simulink model "dual500MHzPFB"  (Simulink 6.2)
settings: Solver=ode45  StartTime=0.0  StopTime=10000  RelTol=1e-3
libraries: xbsIndex_r3 x2070, casper_library x180, xps_library x12, gtkWave x5, gavrt_library x1
(part 11 of 20)

== system dual500MHzPFB/cfgspec/PFB_Subsystem/pfb_fir_real1/pol1_in1_first_tap/pfb_coeff_gen ==
  din : Inport  Port=1  LatchInput=off
  sync : Inport  Port=2  LatchInput=off
  Concat : xbsIndex_r3/Concat  num_inputs=2  explicit_period=off  period=1  dbl_ovrd=off
  Counter : xbsIndex_r3/Counter  cnt_type=Free Running  n_bits=8  bin_pt=0  arith_type=Unsigned  start_count=0  cnt_to=Inf  cnt_by_val=1  operation=Up  explicit_period=on  period=1  load_pin=off  rst=on  en=off  dbl_ovrd=off  show_param=off  use_rpm=on  gen_core=off
      settings: xl_area=[0, 0, 0, 0, 0, 0, 0]
  Delay : xbsIndex_r3/Delay  latency=bram_latency+1  reg_retiming=off  explicit_period=off  period=1  en=off  accept_only_valid=off  init_zero=on  dbl_ovrd=off  show_param=off
      settings: xl_area=[0, 0, 0, 0, 0, 0, 0]
  Delay1 : xbsIndex_r3/Delay  latency=3  reg_retiming=off  explicit_period=off  period=1  en=off  accept_only_valid=off  init_zero=on  dbl_ovrd=off  show_param=off
      settings: xl_area=[0, 0, 0, 0, 0, 0, 0]
  ROM1 : xbsIndex_r3/ROM  depth=256  initVector=[3.1185374660155e-018 0.000313853577146838 0.000630949867739494 0.000952101185429728 0.00127813150918155 0.00160987609990742 0.00194818110908897 0.00229390317955257 0.00264790903857445 0.00301107508349448 0.00338428696002226 0.00376843913342326 0.00416443445277708 0.00457318370850389 0.00499560518335912 0.00543262419710063 0.00588517264503594 0.00635418853066137 0.00684061549260819 0.00734540232611445 0.00786950249924483 0.00841387366408389 0.0089794771631314 0.00956727753113161 0.0101782419925713 0.010813339955084 0.0114735424990016 0.0121598218632949 0.0128731509281507 0.0136145026944319 0.014384849760272 0.0151851637950551 0.0160164150110379 0.0168795716328685 0.0177755993652613 0.0187054608590871 0.0196701151761411 0.0206705172528497 0.0217076173631834 0.0227823605810373 0.023895686242349 0.0250485274072193 0.0262418103223038 0.027476453883745 0.0287533691009129 0.0300734585612245 0.031437615896311 0.0328467252498039 0.0343016607470079 0.0358032859667318 0.0373524534155453 0.0389500040047317 0.0405967665302039 0.042293557155651 0.044041178899183 0.0458404211237378 0.0476920590315163 0.0495968531627079 0.0515555488987685 0.0535688759705108 0.0556375479712659 0.0577622618753727 0.0599436975622499 0.0621825173463032 0.0644793655129179 0.0668348678607861 0.0692496312508128 0.0717242431618448 0.0742592712534627 0.0768552629360733 0.0795127449485372 0.0822322229435622 0.0850141810810928 0.0878590816299174 0.0907673645777188 0.0937394472497809 0.0967757239365713 0.0998765655304047 0.103042319171399 0.106273307902919 0.109569830336718 0.112932160327956 0.116360546660299 0.119855212741273 0.123416356308059 0.127044149143908 0.13073873680534 0.134500238360297 0.138328746137415 0.142224325486561 0.146187014550802 0.15021682404994 0.154313737075755 0.158477708899094 0.162708666788946 0.167006509843603 0.171371108834052 0.175802306059696 0.180299915216515 0.184863721277773 0.189493480387363 0.194188919765877 0.198949737629496 0.203775603121767 0.208666156258342 0.213621007884754 0.218639739647272 0.22372190397691 0.228867024086619 0.234074593981714 0.239344078483567 0.244674913266598 0.250066504908579 0.255518230954276 0.261029439992432 0.266599451746097 0.272227557176302 0.277913018599066 0.283655069815719 0.289452916256518 0.29530573513754 0.301212675630786 0.307172859047495 0.313185379034582 0.31924930178417 0.325363666256144 0.331527484413666 0.33773974147157 0.343999396157563 0.350305380986143 0.356656602545143 0.363051941794802 0.369490254379254 0.375970370950336 0.382491097503579 0.389051215726279 0.395649483357505 0.402284634559911 0.40895538030322 0.415660408759225 0.422398385708151 0.429167954956233 0.435967738764334 0.44279633828744 0.449652334024857 0.456534286280925 0.46344073563607 0.470370203428 0.477321192242848 0.484292186416068 0.491281652542864 0.498288039997961 0.505309781464482 0.512345293471729 0.51939297694163 0.526451217743632 0.533518387257796 0.540592842945872 0.547672928930096 0.55475697657947 0.56184330510328 0.568930222151592 0.576016024422464 0.583098998275629 0.590177420352365 0.597249558201307 0.604313670909903 0.611368009741263 0.61841081877612 0.625440335559606 0.632454791752587 0.639452413787252 0.64643142352668 0.653390038928083 0.660326474709457 0.667238943019316 0.67412565410924 0.68098481700893 0.68781464020346 0.694613332312453 0.701379102770851 0.708110162510993 0.714804724645695 0.721461005152022 0.728077223555458 0.734651603614152 0.741182374002953 0.747667768996907 0.754106029153935 0.760495401996357 0.766834142690977 0.773120514727421 0.779352790594407 0.785529252453665 0.79164819281118 0.797707915185476 0.803706734772626 0.809642979107687 0.815514988722272 0.821321117797946 0.827059734815166 0.832729223197448 0.838327981950501 0.843854426296004 0.849306988299761 0.854684117493933 0.859984281493085 0.865205966603733 0.870347678427156 0.875407942455152 0.880385304658511 0.885278332067902 0.890085613346922 0.894805759357052 0.899437403714244 0.903979203336905 0.908429838985005 ...(+699 chars)]  arith_type="Signed  (2's comp)"  n_bits=8  bin_pt=7  latency=2  init_zero=on  explicit_period=off  period=1  rst=off  init_reg=0  en=off  dbl_ovrd=off  show_param=on  distributed_mem=off  use_rpm=on  gen_core=off
      settings: xl_area=[0, 0, 0, 0, 0, 0, 0]
  ROM2 : xbsIndex_r3/ROM  depth=256  initVector=[0.999999458258868 0.999931021245783 0.999743065596651 0.999435647723483 0.999008859879318 0.998462830120572 0.997797722254753 0.997013735773593 0.996111105771608 0.995090102850134 0.993951033006882 0.992694237511061 0.991320092764127 0.989829010146224 0.988221435848383 0.986497850690571 0.984658769925647 0.982704743029348 0.980636353476378 0.978454218502709 0.976158988854215 0.97375134852174 0.971232014462726 0.968601736309539 0.96586129606462 0.963011507782594 0.960053217239501 0.956987301589287 0.953814669007724 0.950536258323912 0.947153038639539 0.943666008936081 0.940076197670108 0.936384662356893 0.932592489142517 0.928700792364653 0.924710714102252 0.920623423714318 0.916440117367999 0.912162017556199 0.907790372604941 0.903326456170708 0.89877156672798 0.894127027047217 0.889394183663526 0.884574406336234 0.879669087499654 0.874679641705254 0.869607505055511 0.864454134629704 0.859221007901897 0.853909622151394 0.848521493865925 0.843058158137836 0.837521168053561 0.831912094076659 0.826232523424682 0.820484059440178 0.814668320956092 0.80878694165588 0.802841569428602 0.796833865719299 0.790765504874954 0.784638173486316 0.778453569725904 0.77221340268248 0.765919391692288 0.759573265667376 0.753176762421293 0.746731627992459 0.740239615965535 0.733702486791073 0.727122007103769 0.720499949039619 0.713838089552282 0.707138209728965 0.700402094106126 0.693631529985308 0.686828306749403 0.679994215179664 0.673131046773749 0.666240593065125 0.659324644944108 0.65238499198086 0.645423421750641 0.6384417191616 0.63144166578542 0.624425039191102 0.617393612282178 0.610349152637658 0.603293421856988 0.596228174909311 0.589155159487311 0.58207611536593 0.574992773766228 0.567906856724672 0.560820076468121 0.55373413479477 0.546650722461346 0.539571518576789 0.532498190002693 0.525432390760777 0.518375761447603 0.511329928656835 0.504296504409245 0.497277085590735 0.490273253398593 0.483286572796234 0.476318591976636 0.469370841834709 0.462444835448811 0.455542067571624 0.448664014130602 0.441812131738202 0.434987857212088 0.428192607105504 0.421427777248019 0.414694742296809 0.407994855298675 0.401329447262956 0.39469982674551 0.388107279443932 0.381553067804161 0.37503843063862 0.368564582756054 0.362132714603191 0.355743991918358 0.349399555397198 0.343100520370588 0.336847976494894 0.330642987454655 0.324486590677818 0.318379797063608 0.31232359072313 0.306318928732789 0.300366740900606 0.2944679295455 0.288623369289612 0.282833906863717 0.277100360925787 0.271423521892756 0.265804151785514 0.260242984087177 0.254740723614657 0.249298046403554 0.243915599606379 0.238594001404134 0.233333840931226 0.228135678213734 0.22300004412101 0.217927440330587 0.212918339306393 0.207973184290218 0.203092389306419 0.198276339179798 0.193525389566635 0.188839866998784 0.184220068940809 0.179666263860066 0.175178691309668 0.170757562024254 0.166403058028479 0.162115332758128 0.157894511193761 0.153740690006788 0.149653937717859 0.145634294867461 0.141681774198606 0.137796360851467 0.13397801256985 0.130226659919365 0.126542206517129 0.122924529272895 0.119373478641418 0.115888878885919 0.112470528352485 0.10911819975523 0.105831640472054 0.102610572850808 0.0994546945257127 0.0963636787438044 0.0933371747012584 0.0903748078893658 0.0874761804499801 0.0846408715402248 0.0818684377062569 0.0791584132658749 0.0765103106997557 0.0739236210511041 0.0713978143334908 0.0689323399466543 0.0665266271000393 0.0641800852438365 0.0618921045072929 0.0596620561440508 0.0574892929842778 0.0553731498933419 0.0533129442367877 0.0513079763513631 0.0493575300218483 0.0474608729634309 0.045617257309375 0.0438259201037253 0.0420860837987887 0.0403969567571315 0.0387577337578319 0.0371675965067231 0.0356257141503632 0.0341312437934655 0.0326833310195229 0.031281110414359 0.0299237060923366 0.0286102322249562 0.0273397935715735 0.0261114860119683 0.0249243970804927 0.0237776065015307 0.0226701867259983 0.0216012034686154 0.0205697162456796 0.019574778913074 ...(+681 chars)]  arith_type="Signed  (2's comp)"  n_bits=8  bin_pt=7  latency=2  init_zero=on  explicit_period=off  period=1  rst=off  init_reg=0  en=off  dbl_ovrd=off  show_param=on  distributed_mem=off  use_rpm=on  gen_core=off
      settings: xl_area=[0, 0, 0, 0, 0, 0, 0]
  Register : xbsIndex_r3/Register  init=0  reg_only_valid=off  explicit_period=off  period=1  rst=off  en=off  out_en=off  dbl_ovrd=off  show_param=off
      settings: xl_area=[0, 0, 0, 0, 0, 0, 0]
  Reinterpret1 : xbsIndex_r3/Reinterpret  force_arith_type=on  arith_type=Unsigned  force_bin_pt=on  bin_pt=0  force_valid=on
  Reinterpret2 : xbsIndex_r3/Reinterpret  force_arith_type=on  arith_type=Unsigned  force_bin_pt=on  bin_pt=0  force_valid=on
  dout : Outport
  sync_out : Outport  Port=2
  coeff : Outport  Port=3
  wires:
  din/1 -> Delay1/1
  Delay1/1 -> dout/1
  sync/1 -> Counter/1, Delay/1
  Delay/1 -> sync_out/1
  Concat/1 -> Register/1
  Register/1 -> coeff/1
  Counter/1 -> ROM1/1, ROM2/1
  ROM1/1 -> Reinterpret1/1
  Reinterpret1/1 -> Concat/1
  ROM2/1 -> Reinterpret2/1
  Reinterpret2/1 -> Concat/2

== system dual500MHzPFB/cfgspec/PFB_Subsystem/pfb_fir_real1/pol1_in1_last_tap/pfb_real_add_tree ==
  din : Inport  Port=1  LatchInput=off
  sync : Inport  Port=2  LatchInput=off
  Reint0 : xbsIndex_r3/Reinterpret  force_arith_type=on  arith_type="Signed  (2's comp)"  force_bin_pt=on  bin_pt=CoeffBitWidth + BitWidthIn - 2  force_valid=on
  Reint1 : xbsIndex_r3/Reinterpret  force_arith_type=on  arith_type="Signed  (2's comp)"  force_bin_pt=on  bin_pt=CoeffBitWidth + BitWidthIn - 2  force_valid=on
  Slice0 : xbsIndex_r3/Slice  mode=Upper Bit Location + Width  nbits=CoeffBitWidth + BitWidthIn  bit1=-0*(CoeffBitWidth + BitWidthIn)  base1=MSB of Input  bit0=0  base0=MSB of Input  boolean_output=off  explicit_period=off  period=1  dbl_ovrd=off
  Slice1 : xbsIndex_r3/Slice  mode=Upper Bit Location + Width  nbits=CoeffBitWidth + BitWidthIn  bit1=-1*(CoeffBitWidth + BitWidthIn)  base1=MSB of Input  bit0=0  base0=MSB of Input  boolean_output=off  explicit_period=off  period=1  dbl_ovrd=off
  adder_tree1 : Subsystem  AncestorBlock=casper_library/Misc/adder_tree  mask(adder_tree){n_inputs=2, latency=2}
      mask prompts: n_inputs "Number of Inputs"; latency "Add Latency"
      mask help: Sums all inputs using a tree of adds and delays.
      mask init:
      | adder_tree_init(gcb, ...
      |     'n_inputs', n_inputs, ...
      |     'latency', latency);
      settings: AttributesFormatString=latency 2
      mask Help: eval('xlWeb([getenv(''MLIB_ROOT''), ''\doc\html\sp_adder_tree\sp_adder_tree.html''])')
  convert1 : xbsIndex_r3/Convert  arith_type="Signed  (2's comp)"  n_bits=BitWidthOut  bin_pt=BitWidthOut-1  quantization=Truncate  overflow=Saturate  latency=add_latency  explicit_period=off  period=1  dbl_ovrd=off  show_param=off  inserted_by_tool=off  pipeline=off
      settings: xl_area=[0, 0, 0, 0, 0, 0, 0]
  delay1 : xbsIndex_r3/Delay  latency=2  reg_retiming=off  explicit_period=off  period=1  en=off  accept_only_valid=off  init_zero=on  dbl_ovrd=off  show_param=off
      settings: xl_area=[0, 0, 0, 0, 0, 0, 0]
  scale1 : xbsIndex_r3/Scale  scale_factor=-2  explicit_period=off  period=1  dbl_ovrd=off
  dout : Outport
  sync_out : Outport  Port=2
  wires:
  adder_tree1/2(dout) -> scale1/1
  scale1/1 -> convert1/1
  convert1/1 -> dout/1
  sync/1 -> adder_tree1/1(sync)
  adder_tree1/1(sync_out) -> delay1/1
  delay1/1 -> sync_out/1
  din/1 -> Slice0/1, Slice1/1
  Slice0/1 -> Reint0/1
  Reint0/1 -> adder_tree1/2(din1)
  Slice1/1 -> Reint1/1
  Reint1/1 -> adder_tree1/3(din2)

== system dual500MHzPFB/cfgspec/PFB_Subsystem/pfb_fir_real1/pol1_in2_first_tap/delay ==
  In1 : Inport  Port=1  LatchInput=off
  delay_bram : casper_library/Delays/delay_bram  DelayLen=2^(PFBSize-n_inputs)  bram_latency=bram_latency
  Out1 : Outport
  wires:
  In1/1 -> delay_bram/1
  delay_bram/1 -> Out1/1

== system dual500MHzPFB/cfgspec/PFB_Subsystem/pfb_fir_real1/pol1_in2_first_tap/pfb_coeff_gen ==
  din : Inport  Port=1  LatchInput=off
  sync : Inport  Port=2  LatchInput=off
  Concat : xbsIndex_r3/Concat  num_inputs=2  explicit_period=off  period=1  dbl_ovrd=off
  Counter : xbsIndex_r3/Counter  cnt_type=Free Running  n_bits=8  bin_pt=0  arith_type=Unsigned  start_count=0  cnt_to=Inf  cnt_by_val=1  operation=Up  explicit_period=on  period=1  load_pin=off  rst=on  en=off  dbl_ovrd=off  show_param=off  use_rpm=on  gen_core=off
      settings: xl_area=[0, 0, 0, 0, 0, 0, 0]
  Delay : xbsIndex_r3/Delay  latency=bram_latency+1  reg_retiming=off  explicit_period=off  period=1  en=off  accept_only_valid=off  init_zero=on  dbl_ovrd=off  show_param=off
      settings: xl_area=[0, 0, 0, 0, 0, 0, 0]
  Delay1 : xbsIndex_r3/Delay  latency=3  reg_retiming=off  explicit_period=off  period=1  en=off  accept_only_valid=off  init_zero=on  dbl_ovrd=off  show_param=off
      settings: xl_area=[0, 0, 0, 0, 0, 0, 0]
  ROM1 : xbsIndex_r3/ROM  depth=256  initVector=[7.82033640873917e-005 0.000392792117321438 0.00071082554813207 0.00103311892199487 0.00136049907461725 0.00169380402655518 0.00203388258985642 0.00238159396690193 0.00273780734162119 0.00310340146326166 0.00347926422289714 0.00386629222286377 0.00426539033931678 0.00467747127810509 0.00510345512416486 0.00554426888463693 0.00600084602591724 0.00647412600485223 0.00696505379429587 0.00747457940324748 0.00800365739179369 0.00855324638108065 0.00912430855854599 0.00971780917864314 0.0103347160592936 0.0109759990743052 0.0116426296419981 0.0123355802102817 0.0130558237384286 0.0138043331757953 0.0145820809377384 0.0153900383789824 0.0162291752646908 0.0171004592395002 0.0180048552947743 0.0189433252343389 0.0199168271389599 0.0209263148298273 0.021972737331309 0.0230570383332419 0.0241801556530246 0.0253430206977808 0.0265465579268609 0.0277916843149512 0.0290793088160584 0.0304103318286413 0.0317856446621574 0.0332061290052946 0.0346726563961596 0.0361860876946888 0.0377472725575551 0.0393570489158354 0.0410162424557095 0.0427256661024564 0.0444861195080145 0.046298388542371 0.0481632447890453 0.0500814450449274 0.0520537308247352 0.0540808278703483 0.0561634456652778 0.0583022769545272 0.0604979972700995 0.0627512644624029 0.0650627182378034 0.067432979702574 0.0698626509134837 0.07235231443527 0.0749025329052334 0.0775138486051921 0.0801867830410294 0.082921836530065 0.0857194877964775 0.0885801935750023 0.0915043882231255 0.0944924833419901 0.0975448674062286 0.100661905402931 0.103843938479953 0.107091283603769 0.110404233227058 0.113783054966233 0.117227991289079 0.120739259212706 0.124317050011981 0.127961528938623 0.131672834951122 0.135451080455663 0.139296351058194 0.143208705327813 0.147188174571609 0.151234762621111 0.155348445630488 0.159529171886614 0.163776861631156 0.168091406894782 0.172472671343625 0.176920490138103 0.18143466980421 0.186014988117371 0.190661193998959 0.195373007425566 0.200150119351105 0.204992191641821 0.209898857024285 0.214869719046434 0.219904352051709 0.225002301166354 0.230163082299916 0.235386182158984 0.240671058274206 0.2460171390406 0.251423823771201 0.256890482764031 0.262416457382418 0.26800106014867 0.273643574851073 0.279343256664236 0.285099332282737 0.290911000068066 0.296777430208813 0.302697764894093 0.308671118500132 0.314696577789995 0.320773202126374 0.326900023697389 0.333076047755331 0.339300252868267 0.345571591184427 0.351888988709288 0.358251345595259 0.364657536443868 0.37110641062034 0.377596792580462 0.384127482209607 0.390697255173799 0.397304863282687 0.40394903486429 0.41062847515137 0.417341866679289 0.424087869695195 0.430865122578368 0.437672242271578 0.444507824723272 0.451370445340415 0.458258659451806 0.46517100278169 0.472105991933451 0.479062124883217 0.486037881483159 0.493031723974274 0.50004209750845 0.507067430679598 0.514106136063612 0.521156610766955 0.528217236983621 0.535286382560249 0.542362401569151 0.549443634889005 0.556528410792964 0.563615045543947 0.570701843996833 0.577787100207321 0.584869098047179 0.591946111825632 0.599016406916601 0.606078240391542 0.613129861657594 0.620169513100771 0.627195430733905 0.634205844849072 0.641198980674199 0.648173059033581 0.655126297012004 0.662056908622189 0.668963105475262 0.675843097453958 0.682695093388247 0.6895173017331 0.696307931248092 0.703065191678525 0.709787294437785 0.716472453290627 0.723118885037072 0.729724810196624 0.736288453692496 0.742808045535534 0.749281821507542 0.755708023843698 0.762084901913749 0.768410712901686 0.774683722483594 0.780902205503364 0.787064446645969 0.793168741108002 0.799213395265163 0.805196727336407 0.811117068044443 0.816972761272283 0.822762164715558 0.828483650530292 0.834135605975834 0.839716434052685 0.84522455413489 0.850658402596745 0.856016433433509 0.861297118875845 0.866498949997721 0.871620437317469 0.876660111391761 0.881616523402199 0.886488245734271 0.891273872548405 0.89597202034285 0.900581328508143 0.905100459872888 0.909528101240623 ...(+701 chars)]  arith_type="Signed  (2's comp)"  n_bits=8  bin_pt=7  latency=2  init_zero=on  explicit_period=off  period=1  rst=off  init_reg=0  en=off  dbl_ovrd=off  show_param=on  distributed_mem=off  use_rpm=on  gen_core=off
      settings: xl_area=[0, 0, 0, 0, 0, 0, 0]
  ROM2 : xbsIndex_r3/ROM  depth=256  initVector=[0.999993555614484 0.999895235614821 0.999677407720508 0.999340137306542 0.99888352558091 0.998307709543272 0.997612861929031 0.996799191138817 0.995866941153415 0.994816391434173 0.993647856808947 0.992361687343622 0.99095826819928 0.989438019475073 0.987801396036875 0.986048887331801 0.984181017188665 0.982198343604478 0.980101458517079 0.977890987564016 0.975567589827767 0.973131957567446 0.970584815937088 0.967926922690669 0.965159067873983 0.962282073503518 0.959296793232491 0.956204112004174 0.953004945692698 0.949700240731477 0.946290973729442 0.942778151075241 0.939162808529609 0.935446010806083 0.931628851140254 0.927712450847762 0.923697958871232 0.919586551316358 0.915379430977356 0.911077826851989 0.906682993646407 0.902196211270012 0.897618784320587 0.892952041559925 0.888197335380202 0.883356041261322 0.878429557219512 0.873419303247388 0.868326720745771 0.863153271947495 0.857900439333497 0.852569725041413 0.847162650267003 0.841680754658628 0.83612559570509 0.830498748117097 0.824801803202644 0.819036368236582 0.813204065824676 0.807306533262431 0.801345421888981 0.795322396436338 0.789239134374282 0.783097325251212 0.776898670031231 0.770644880427786 0.764337678234152 0.757978794651064 0.751569969611804 0.745112951105048 0.738609494495772 0.732061361844525 0.725470321225382 0.718838146042869 0.71216661434818 0.705457508154989 0.698712612755152 0.691933716034627 0.685122607789892 0.678281079045185 0.671410921370864 0.66451392620319 0.657591884165825 0.65064658439337 0.643679813857221 0.636693356694045 0.629688993537183 0.622668500851263 0.615633650270321 0.608586207939725 0.601527933862177 0.594460581248096 0.587385895870655 0.580305615425757 0.573221468897224 0.566135175927489 0.55904844619404 0.551962978791909 0.544880461622458 0.537802570788727 0.530730969997615 0.52366730996913 0.516613227852975 0.509570346652719 0.502540274657783 0.495524604883502 0.488524914519479 0.481542764386477 0.474579698402069 0.467637243055272 0.460716906890385 0.453820180000238 0.446948533529066 0.440103419185214 0.433286268763866 0.426498493679995 0.419741484511721 0.413016610554267 0.406325219384677 0.399668636437484 0.393048164591489 0.386465083767804 0.379920650539333 0.373416097751825 0.366952634156649 0.360531444055436 0.354153686956706 0.347820497244626 0.34153298386 0.335292229993622 0.329099292792089 0.322955203076182 0.316860965071917 0.310817556154338 0.304825926604156 0.2988869993773 0.293001669887455 0.287170805801649 0.281395246848952 0.275675804642333 0.270013262513728 0.264408375362351 0.258861869516288 0.253374442607394 0.247946763459516 0.242579471990057 0.237273179124887 0.232028466726598 0.226845887536105 0.221725965127573 0.21666919387666 0.211676038942041 0.206746936260191 0.201882292553387 0.197082485350882 0.192347863023202 0.187678744829518 0.183075420978016 0.178538152699211 0.174067172332122 0.169662683423225 0.165324860838114 0.161053850885749 0.156849771455227 0.152712712164937 0.148642734524024 0.144639872106008 0.14070413073448 0.136835488680706 0.133033896873036 0.129299279117972 0.125631532332744 0.12203052678926 0.118496106369262 0.115028088830537 0.111626266084031 0.108290404481666 0.105020245114723 0.101815504122587 0.0986758730116877 0.0956010189844369 0.0925905852779795 0.0896441915125591 0.0867614340492978 0.0839418863571882 0.0811850993890874 0.0784906019665026 0.0758579011729519 0.0732864827556818 0.0707758115355173 0.0683253318246198 0.0659344678519223 0.0636026241960095 0.0613291862252073 0.0591135205446423 0.056954975450031 0.0548528813879534 0.0528065514223651 0.0508152817070987 0.0488783519641021 0.0469950259671621 0.0451645520308558 0.0433861635044739 0.0416590792706549 0.0399825042484717 0.0383556299007058 0.0367776347450473 0.0352476848689546 0.0337649344479084 0.0323285262667932 0.0309375922441371 0.029591253958944 0.0282886231798464 0.0270288023963116 0.0258108853516301 0.0246339575774173 0.0234970969293587 0.0223993741239277 0.0213398532758088 0.0203175924357544 ...(+708 chars)]  arith_type="Signed  (2's comp)"  n_bits=8  bin_pt=7  latency=2  init_zero=on  explicit_period=off  period=1  rst=off  init_reg=0  en=off  dbl_ovrd=off  show_param=on  distributed_mem=off  use_rpm=on  gen_core=off
      settings: xl_area=[0, 0, 0, 0, 0, 0, 0]
  Register : xbsIndex_r3/Register  init=0  reg_only_valid=off  explicit_period=off  period=1  rst=off  en=off  out_en=off  dbl_ovrd=off  show_param=off
      settings: xl_area=[0, 0, 0, 0, 0, 0, 0]
  Reinterpret1 : xbsIndex_r3/Reinterpret  force_arith_type=on  arith_type=Unsigned  force_bin_pt=on  bin_pt=0  force_valid=on
  Reinterpret2 : xbsIndex_r3/Reinterpret  force_arith_type=on  arith_type=Unsigned  force_bin_pt=on  bin_pt=0  force_valid=on
  dout : Outport
  sync_out : Outport  Port=2
  coeff : Outport  Port=3
  wires:
  din/1 -> Delay1/1
  Delay1/1 -> dout/1
  sync/1 -> Counter/1, Delay/1
  Delay/1 -> sync_out/1
  Concat/1 -> Register/1
  Register/1 -> coeff/1
  Counter/1 -> ROM1/1, ROM2/1
  ROM1/1 -> Reinterpret1/1
  Reinterpret1/1 -> Concat/1
  ROM2/1 -> Reinterpret2/1
  Reinterpret2/1 -> Concat/2

== system dual500MHzPFB/cfgspec/PFB_Subsystem/pfb_fir_real1/pol1_in2_last_tap/pfb_real_add_tree ==
  din : Inport  Port=1  LatchInput=off
  sync : Inport  Port=2  LatchInput=off
  Reint0 : xbsIndex_r3/Reinterpret  force_arith_type=on  arith_type="Signed  (2's comp)"  force_bin_pt=on  bin_pt=CoeffBitWidth + BitWidthIn - 2  force_valid=on
  Reint1 : xbsIndex_r3/Reinterpret  force_arith_type=on  arith_type="Signed  (2's comp)"  force_bin_pt=on  bin_pt=CoeffBitWidth + BitWidthIn - 2  force_valid=on
  Slice0 : xbsIndex_r3/Slice  mode=Upper Bit Location + Width  nbits=CoeffBitWidth + BitWidthIn  bit1=-0*(CoeffBitWidth + BitWidthIn)  base1=MSB of Input  bit0=0  base0=MSB of Input  boolean_output=off  explicit_period=off  period=1  dbl_ovrd=off
  Slice1 : xbsIndex_r3/Slice  mode=Upper Bit Location + Width  nbits=CoeffBitWidth + BitWidthIn  bit1=-1*(CoeffBitWidth + BitWidthIn)  base1=MSB of Input  bit0=0  base0=MSB of Input  boolean_output=off  explicit_period=off  period=1  dbl_ovrd=off
  adder_tree1 : Subsystem  AncestorBlock=casper_library/Misc/adder_tree  mask(adder_tree){n_inputs=2, latency=2}
      mask prompts: n_inputs "Number of Inputs"; latency "Add Latency"
      mask help: Sums all inputs using a tree of adds and delays.
      mask init:
      | adder_tree_init(gcb, ...
      |     'n_inputs', n_inputs, ...
      |     'latency', latency);
      settings: AttributesFormatString=latency 2
      mask Help: eval('xlWeb([getenv(''MLIB_ROOT''), ''\doc\html\sp_adder_tree\sp_adder_tree.html''])')
  convert1 : xbsIndex_r3/Convert  arith_type="Signed  (2's comp)"  n_bits=BitWidthOut  bin_pt=BitWidthOut-1  quantization=Truncate  overflow=Saturate  latency=add_latency  explicit_period=off  period=1  dbl_ovrd=off  show_param=off  inserted_by_tool=off  pipeline=off
      settings: xl_area=[0, 0, 0, 0, 0, 0, 0]
  delay1 : xbsIndex_r3/Delay  latency=2  reg_retiming=off  explicit_period=off  period=1  en=off  accept_only_valid=off  init_zero=on  dbl_ovrd=off  show_param=off
      settings: xl_area=[0, 0, 0, 0, 0, 0, 0]
  scale1 : xbsIndex_r3/Scale  scale_factor=-2  explicit_period=off  period=1  dbl_ovrd=off
  dout : Outport
  sync_out : Outport  Port=2
  wires:
  adder_tree1/2(dout) -> scale1/1
  scale1/1 -> convert1/1
  convert1/1 -> dout/1
  sync/1 -> adder_tree1/1(sync)
  adder_tree1/1(sync_out) -> delay1/1
  delay1/1 -> sync_out/1
  din/1 -> Slice0/1, Slice1/1
  Slice0/1 -> Reint0/1
  Reint0/1 -> adder_tree1/2(din1)
  Slice1/1 -> Reint1/1
  Reint1/1 -> adder_tree1/3(din2)

== system dual500MHzPFB/cfgspec/PFB_Subsystem/pfb_fir_real1/pol1_in3_first_tap/delay ==
  In1 : Inport  Port=1  LatchInput=off
  delay_bram : casper_library/Delays/delay_bram  DelayLen=2^(PFBSize-n_inputs)  bram_latency=bram_latency
  Out1 : Outport
  wires:
  In1/1 -> delay_bram/1
  delay_bram/1 -> Out1/1

== system dual500MHzPFB/cfgspec/PFB_Subsystem/pfb_fir_real1/pol1_in3_first_tap/pfb_coeff_gen ==
  din : Inport  Port=1  LatchInput=off
  sync : Inport  Port=2  LatchInput=off
  Concat : xbsIndex_r3/Concat  num_inputs=2  explicit_period=off  period=1  dbl_ovrd=off
  Counter : xbsIndex_r3/Counter  cnt_type=Free Running  n_bits=8  bin_pt=0  arith_type=Unsigned  start_count=0  cnt_to=Inf  cnt_by_val=1  operation=Up  explicit_period=on  period=1  load_pin=off  rst=on  en=off  dbl_ovrd=off  show_param=off  use_rpm=on  gen_core=off
      settings: xl_area=[0, 0, 0, 0, 0, 0, 0]
  Delay : xbsIndex_r3/Delay  latency=bram_latency+1  reg_retiming=off  explicit_period=off  period=1  en=off  accept_only_valid=off  init_zero=on  dbl_ovrd=off  show_param=off
      settings: xl_area=[0, 0, 0, 0, 0, 0, 0]
  Delay1 : xbsIndex_r3/Delay  latency=3  reg_retiming=off  explicit_period=off  period=1  en=off  accept_only_valid=off  init_zero=on  dbl_ovrd=off  show_param=off
      settings: xl_area=[0, 0, 0, 0, 0, 0, 0]
  ROM1 : xbsIndex_r3/ROM  depth=256  initVector=[0.000156571753004131 0.000471945891501983 0.000790967418464927 0.00111445452761384 0.00144323688731232 0.0017781552531742 0.00212006107274008 0.0024698160823956 0.00282829189670815 0.00319636959036365 0.00357493927288892 0.00396489965634961 0.00436715761621773 0.00478262774560706 0.00521223190307826 0.00565689875421988 0.00611756330721485 0.006595166442606 0.0070906544374775 0.00760497848427273 0.00813909420447243 0.00869396115736018 0.00927054234410557 0.00986980370739833 0.0104927136268696 0.0111402424105394 0.0118133617825326 0.0125130443673066 0.0132402631706387 0.013995991057622 0.0147812002279213 0.0155968616885416 0.016443944724367 0.0173234163667243 0.0182362408602338 0.0191833791282049 0.0201657882368408 0.0211844208585156 0.0222402247343869 0.0233341421366126 0.0244671093304362 0.0256400560364093 0.0268539048930204 0.028109570919997 0.0294079609825521 0.0307499732568442 0.0321364966969199 0.0335684105034094 0.0350465835942454 0.0365718740776727 0.03814512872782 0.0397671824631001 0.0414388578277084 0.0431609644764848 0.0449342986634068 0.0467596427339775 0.0486377646217729 0.0505694173494113 0.0525553385342047 0.0545962498987528 0.0566928567867364 0.0588458476841667 0.0610558937463428 0.0633236483307712 0.0656497465362942 0.0680348047486762 0.0704794201928911 0.0729841704923531 0.0755496132353287 0.0781762855487681 0.080864703679787 0.0836153625850295 0.0864287355281387 0.0893052736855576 0.0922454057608818 0.0952495376079764 0.0983180518630736 0.101451307586057 0.104649639911135 0.107913359707113 0.111242753247444 0.114638081890267 0.118099581768609 0.121627463490941 0.125221911852256 0.128883085555861 0.132611116946024 0.136406111751676 0.140268148841289 0.144197279989117 0.148193529652922 0.152256894763353 0.156387344525091 0.160584820229917 0.164849235081815 0.169180474034232 0.173578393639624 0.178042821911379 0.182573558198244 0.187170373071336 0.191833008223839 0.196561176383476 0.201354561237828 0.206212817372591 0.211135570222817 0.216122416037231 0.22117292185565 0.226286625499582 0.231463035576027 0.236701631494537 0.242001863497553 0.247363152704048 0.252784891166504 0.258266441941216 0.263807139171958 0.269406288186976 0.275063165609337 0.280777019480592 0.286547069397754 0.292372506663552 0.298252494449934 0.304186167974785 0.310172634691807 0.316210974493512 0.322300239927273 0.328439456424369 0.334627622541945 0.340863710217824 0.347146665038078 0.353475406517269 0.359848828391271 0.36626579892256 0.372725161217884 0.379225733558168 0.385766309740569 0.392345659432526 0.398962528537691 0.405615639573596 0.412303692060908 0.419025362924137 0.425779306903621 0.432564156978649 0.439378524801535 0.446221001142489 0.453090156345094 0.459984540792213 0.466902685382136 0.473843102014779 0.48080428408772 0.487784707001898 0.49478282867673 0.501797090074468 0.508825915733558 0.515867714310774 0.522920879131923 0.529983788750869 0.537054807516645 0.54413228614842 0.551214562318069 0.558299961240106 0.565386796268718 0.572473369501655 0.579557972390709 0.586638886358525 0.593714383421474 0.600782726818319 0.607842171644411 0.614890965491117 0.62192734909023 0.628949556963061 0.635955818073934 0.642944356487798 0.649913392031675 0.656861140959638 0.663785816621042 0.670685630131702 0.677558791047733 0.684403508041737 0.691217989581062 0.698000444607801 0.704749083220269 0.711462117355605 0.718137761473247 0.724774233238938 0.731369754208968 0.737922550514358 0.744430853544664 0.750892900631098 0.757306935728673 0.763671210097042 0.769983982979752 0.776243522281579 0.782448105243668 0.788596019116149 0.794685561827938 0.800715042653424 0.806682782875726 0.812587116446239 0.818426390640147 0.824198966707636 0.829903220520478 0.835537543213724 0.84110034182219 0.846590039911459 0.852005078203117 0.85734391519392 0.862605027768629 0.867786911806227 0.872888082779229 0.87790707634584 0.88284244893466 0.887692778321693 0.892456664199373 0.897132728737377 0.901719617134936 0.90621599816441 0.910620564705884 ...(+696 chars)]  arith_type="Signed  (2's comp)"  n_bits=8  bin_pt=7  latency=2  init_zero=on  explicit_period=off  period=1  rst=off  init_reg=0  en=off  dbl_ovrd=off  show_param=on  distributed_mem=off  use_rpm=on  gen_core=off
      settings: xl_area=[0, 0, 0, 0, 0, 0, 0]
  ROM2 : xbsIndex_r3/ROM  depth=256  initVector=[0.999980181706812 0.999851980565338 0.999604284511911 0.999237167882849 0.998750740838502 0.998145149318279 0.99742057498107 0.996577235131088 0.995615382629159 0.994535305789518 0.993337328262134 0.99202180890064 0.990589141615924 0.989039755215435 0.987374113228298 0.985592713716306 0.983696089070883 0.981684805796099 0.979559464277863 0.97732069853937 0.974969175982937 0.972505597118337 0.969930695277763 0.967245236317542 0.96445001830675 0.961545871202867 0.958533656514614 0.955414266952141 0.952188626064713 0.948857687866076 0.945422436447659 0.941883885579808 0.938243078301218 0.934501086496762 0.93065901046392 0.926717978467979 0.922679146286243 0.918543696741437 0.914312839224529 0.909987809207196 0.905569867744142 0.901060300965507 0.896460419559603 0.891771558246203 0.886995075240635 0.882132351708915 0.877184791214188 0.872153819154706 0.867040882193617 0.86184744768082 0.856575003067155 0.851225055311182 0.845799130278843 0.840298772136253 0.83472554273592 0.829081020996665 0.823366802277519 0.817584497745891 0.811735733740289 0.805822151127884 0.799845404657212 0.793807162306308 0.787709104626554 0.781552924082562 0.775340324388371 0.76907301984027 0.762752734646535 0.756381202254406 0.749960164674578 0.743491371803535 0.736976580744021 0.730417555123955 0.723816064414095 0.71717388324476 0.710492790721915 0.703774569742931 0.697021006312307 0.690233888857689 0.683415007546466 0.676566153603261 0.669689118628614 0.662785693919171 0.655857669789663 0.648906834896993 0.641934975566721 0.634943875122243 0.627935313216969 0.620911065169787 0.613872901304108 0.606822586290777 0.599761878495151 0.592692529328615 0.585616282604827 0.578534873900973 0.571450029924306 0.56436346788425 0.557276894870328 0.550192007236204 0.543110489990084 0.536034016191747 0.528964246356468 0.521902827866082 0.514851394387443 0.507811565298521 0.500784945122391 0.493773122969342 0.486777671987345 0.479800148821113 0.472842093079979 0.465905026814805 0.458990454004159 0.452099860049946 0.445234711282726 0.438396454476901 0.431586516375986 0.424806303228137 0.418057200332153 0.411340571594091 0.40465775909472 0.398010082667942 0.391398839490374 0.384825303682239 0.378290725919721 0.371796333058942 0.365343327771685 0.358932888193021 0.352566167580962 0.34624429398826 0.33996836994648 0.333739472162456 0.32755865122724 0.321426931337641 0.31534531003045 0.309314757929439 0.303336218505222 0.297410607848047 0.291538814453586 0.2857216990218 0.279960094268917 0.274254804752596 0.268606606710293 0.263016247910897 0.257484447519645 0.252011895976347 0.246599254886948 0.241247156928422 0.235956205767024 0.230726975989882 0.225560013049927 0.220455833224157 0.215414923585196 0.210437741986143 0.205524717058656 0.20067624822426 0.195892705718796 0.191174430630003 0.18652173494814 0.181934901629597 0.177414184673436 0.172959809210765 0.168571971606878 0.164250839576072 0.159996552309034 0.155809220612716 0.151688927062585 0.147635726167125 0.143649644544501 0.139730681111232 0.135878807282765 0.132093967185811 0.128376077882305 0.124725029604834 0.121140686003409 0.117622884403397 0.114171436074477 0.110786126510436 0.107466715719658 0.104212938526102 0.101024504880621 0.0979011001824149 0.0948423856104419 0.0918479984645913 0.088917552516421 0.0860506383692603 0.083246823827471 0.0805056542746607 0.0778266530606313 0.0752093218968506 0.0726531412602235 0.0701575708049404 0.0677220497821762 0.0653459974674089 0.0630288135951235 0.0607698788006672 0.0585685550690139 0.0564241861901975 0.054336098221168 0.0523035999538251 0.0503259833889764 0.048402524215972 0.0465324822977585 0.0447151021610977 0.0429496134916917 0.0412352316339554 0.0395711580951738 0.0379565810537831 0.0363906758715103 0.0348726056091064 0.0334015215454071 0.0319765636994546 0.0305968613554102 0.0292615335899919 0.0279696898021663 0.0267204302448249 0.0255128465581769 0.0243460223045864 0.0232190335045865 0.0221309491737983 0.0210808318604881 0.0200677381834912 0.0190907193702359 ...(+687 chars)]  arith_type="Signed  (2's comp)"  n_bits=8  bin_pt=7  latency=2  init_zero=on  explicit_period=off  period=1  rst=off  init_reg=0  en=off  dbl_ovrd=off  show_param=on  distributed_mem=off  use_rpm=on  gen_core=off
      settings: xl_area=[0, 0, 0, 0, 0, 0, 0]
  Register : xbsIndex_r3/Register  init=0  reg_only_valid=off  explicit_period=off  period=1  rst=off  en=off  out_en=off  dbl_ovrd=off  show_param=off
      settings: xl_area=[0, 0, 0, 0, 0, 0, 0]
  Reinterpret1 : xbsIndex_r3/Reinterpret  force_arith_type=on  arith_type=Unsigned  force_bin_pt=on  bin_pt=0  force_valid=on
  Reinterpret2 : xbsIndex_r3/Reinterpret  force_arith_type=on  arith_type=Unsigned  force_bin_pt=on  bin_pt=0  force_valid=on
  dout : Outport
  sync_out : Outport  Port=2
  coeff : Outport  Port=3
  wires:
  din/1 -> Delay1/1
  Delay1/1 -> dout/1
  sync/1 -> Counter/1, Delay/1
  Delay/1 -> sync_out/1
  Concat/1 -> Register/1
  Register/1 -> coeff/1
  Counter/1 -> ROM1/1, ROM2/1
  ROM1/1 -> Reinterpret1/1
  Reinterpret1/1 -> Concat/1
  ROM2/1 -> Reinterpret2/1
  Reinterpret2/1 -> Concat/2

== system dual500MHzPFB/cfgspec/PFB_Subsystem/pfb_fir_real1/pol1_in3_last_tap/pfb_real_add_tree ==
  din : Inport  Port=1  LatchInput=off
  sync : Inport  Port=2  LatchInput=off
  Reint0 : xbsIndex_r3/Reinterpret  force_arith_type=on  arith_type="Signed  (2's comp)"  force_bin_pt=on  bin_pt=CoeffBitWidth + BitWidthIn - 2  force_valid=on
  Reint1 : xbsIndex_r3/Reinterpret  force_arith_type=on  arith_type="Signed  (2's comp)"  force_bin_pt=on  bin_pt=CoeffBitWidth + BitWidthIn - 2  force_valid=on
  Slice0 : xbsIndex_r3/Slice  mode=Upper Bit Location + Width  nbits=CoeffBitWidth + BitWidthIn  bit1=-0*(CoeffBitWidth + BitWidthIn)  base1=MSB of Input  bit0=0  base0=MSB of Input  boolean_output=off  explicit_period=off  period=1  dbl_ovrd=off
  Slice1 : xbsIndex_r3/Slice  mode=Upper Bit Location + Width  nbits=CoeffBitWidth + BitWidthIn  bit1=-1*(CoeffBitWidth + BitWidthIn)  base1=MSB of Input  bit0=0  base0=MSB of Input  boolean_output=off  explicit_period=off  period=1  dbl_ovrd=off
  adder_tree1 : Subsystem  AncestorBlock=casper_library/Misc/adder_tree  mask(adder_tree){n_inputs=2, latency=2}
      mask prompts: n_inputs "Number of Inputs"; latency "Add Latency"
      mask help: Sums all inputs using a tree of adds and delays.
      mask init:
      | adder_tree_init(gcb, ...
      |     'n_inputs', n_inputs, ...
      |     'latency', latency);
      settings: AttributesFormatString=latency 2
      mask Help: eval('xlWeb([getenv(''MLIB_ROOT''), ''\doc\html\sp_adder_tree\sp_adder_tree.html''])')
  convert1 : xbsIndex_r3/Convert  arith_type="Signed  (2's comp)"  n_bits=BitWidthOut  bin_pt=BitWidthOut-1  quantization=Truncate  overflow=Saturate  latency=add_latency  explicit_period=off  period=1  dbl_ovrd=off  show_param=off  inserted_by_tool=off  pipeline=off
      settings: xl_area=[0, 0, 0, 0, 0, 0, 0]
  delay1 : xbsIndex_r3/Delay  latency=2  reg_retiming=off  explicit_period=off  period=1  en=off  accept_only_valid=off  init_zero=on  dbl_ovrd=off  show_param=off
      settings: xl_area=[0, 0, 0, 0, 0, 0, 0]
  scale1 : xbsIndex_r3/Scale  scale_factor=-2  explicit_period=off  period=1  dbl_ovrd=off
  dout : Outport
  sync_out : Outport  Port=2
  wires:
  adder_tree1/2(dout) -> scale1/1
  scale1/1 -> convert1/1
  convert1/1 -> dout/1
  sync/1 -> adder_tree1/1(sync)
  adder_tree1/1(sync_out) -> delay1/1
  delay1/1 -> sync_out/1
  din/1 -> Slice0/1, Slice1/1
  Slice0/1 -> Reint0/1
  Reint0/1 -> adder_tree1/2(din1)
  Slice1/1 -> Reint1/1
  Reint1/1 -> adder_tree1/3(din2)

== system dual500MHzPFB/cfgspec/PFB_Subsystem/pfb_fir_real1/pol1_in4_first_tap/delay ==
  In1 : Inport  Port=1  LatchInput=off
  delay_bram : casper_library/Delays/delay_bram  DelayLen=2^(PFBSize-n_inputs)  bram_latency=bram_latency
  Out1 : Outport
  wires:
  In1/1 -> delay_bram/1
  delay_bram/1 -> Out1/1
